simulink model "MGietka_3"  (R2020b)
settings: Solver=VariableStepAuto  StartTime=0.0  StopTime=10.0  RelTol=1e-3
undefined symbols (not defined in the file): A, B, C, K, N
libraries: simulink x2
settings Model: Creator=Mati  LastModifiedBy=Mati

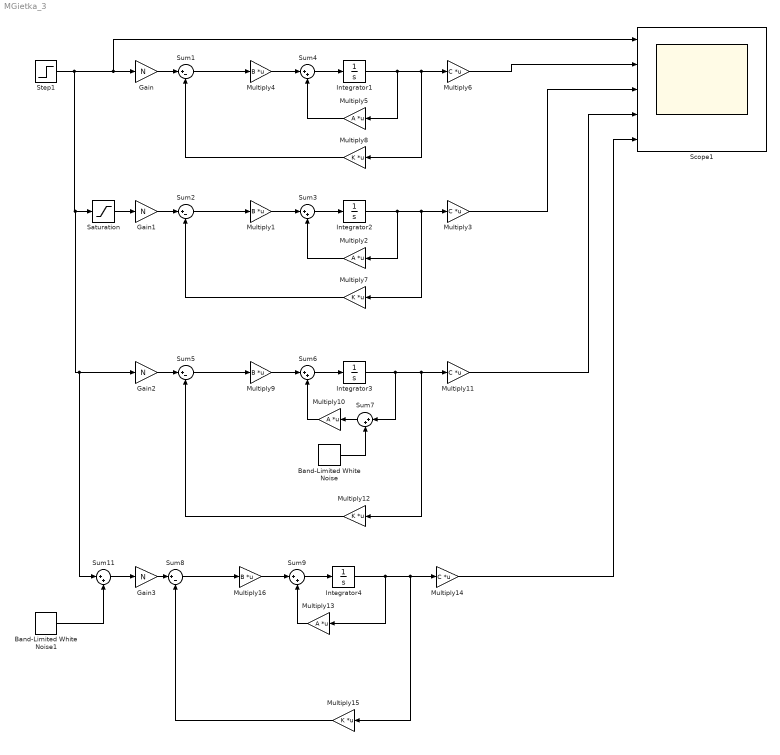
== system MGietka_3 ==
  Band-Limited White Noise : simulink/Sources/Band-Limited White Noise  Cov=[0.0001]  Ts=0.1  seed=[23341]
  Band-Limited White Noise1 : simulink/Sources/Band-Limited White Noise  Cov=[0.0001]  Ts=0.1  seed=[23341]
  Gain{,1..3} (4 alike) : Gain  Gain=N
  Integrator{1..4} (4 alike) : Integrator
  Multiply{1,4,9,16} (4 alike) : Gain  Gain=B  Multiplication=Matrix(K*u)
  Multiply{2,5,10,13} (4 alike) : Gain  Gain=A  Multiplication=Matrix(K*u)
  Multiply{3,6,11,14} (4 alike) : Gain  Gain=C  Multiplication=Matrix(K*u)
  Multiply{7..8,12,15} (4 alike) : Gain  Gain=K  Multiplication=Matrix(K*u)
  Saturation : Saturate  UpperLimit=0.6  LowerLimit=-0.6
  Scope1 : Scope  NumInputPorts=5
  Step1 : Step  SampleTime=0
  Sum{1..2,5,8} (4 alike) : Sum  Inputs=|+-
  Sum{3..4,6..7,9,11} (6 alike) : Sum  Inputs=|++
  wires:
  Gain/1 -> Sum1/1
  Integrator1/1 -> Multiply5/1, Multiply8/1, Multiply6/1
  Multiply8/1 -> Sum1/2
  Multiply4/1 -> Sum4/1
  Sum1/1 -> Multiply4/1
  Multiply5/1 -> Sum4/2
  Sum4/1 -> Integrator1/1
  Multiply6/1 -> Scope1/2
  Multiply7/1 -> Sum2/2
  Sum2/1 -> Multiply1/1
  Multiply1/1 -> Sum3/1
  Integrator2/1 -> Multiply2/1, Multiply7/1, Multiply3/1
  Gain1/1 -> Sum2/1
  Multiply2/1 -> Sum3/2
  Sum3/1 -> Integrator2/1
  Multiply3/1 -> Scope1/3
  Saturation/1 -> Gain1/1
  Step1/1 -> Sum11/1, Gain2/1, Saturation/1, Gain/1, Scope1/1
  Gain2/1 -> Sum5/1
  Multiply10/1 -> Sum6/2
  Integrator3/1 -> Sum7/1, Multiply12/1, Multiply11/1
  Sum6/1 -> Integrator3/1
  Multiply12/1 -> Sum5/2
  Sum5/1 -> Multiply9/1
  Multiply9/1 -> Sum6/1
  Multiply11/1 -> Scope1/4
  Sum7/1 -> Multiply10/1
  Band-Limited White Noise/1 -> Sum7/2
  Gain3/1 -> Sum8/1
  Multiply15/1 -> Sum8/2
  Sum8/1 -> Multiply16/1
  Integrator4/1 -> Multiply13/1, Multiply15/1, Multiply14/1
  Multiply13/1 -> Sum9/2
  Sum9/1 -> Integrator4/1
  Multiply16/1 -> Sum9/1
  Sum11/1 -> Gain3/1
  Band-Limited White Noise1/1 -> Sum11/2
  Multiply14/1 -> Scope1/5
